simulink model "Question_2"  (R2021a)
settings: Solver=VariableStepAuto  StartTime=0.0  StopTime=10.0  RelTol=1e-3
settings Model: Creator=haden  LastModifiedBy=haden

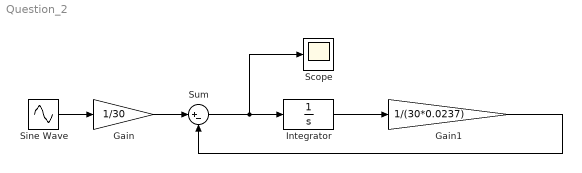
== system Question_2 ==
  Gain : Gain  Gain=1/30
  Gain1 : Gain  Gain=1/(30*0.0237)
  Integrator : Integrator
  Scope : Scope
  Sine Wave : Sin  Amplitude=.1  Frequency=2*pi  SampleTime=0
  Sum : Sum  Inputs=|+-
  wires:
  Gain/1 -> Sum/1
  Sum/1 -> Scope/1, Integrator/1
  Integrator/1 -> Gain1/1
  Gain1/1 -> Sum/2
  Sine Wave/1 -> Gain/1
